simulink model "third"  (R2021b)
settings: Solver=VariableStepAuto  StartTime=0.0  StopTime=30.0  RelTol=1e-3
values from neighbouring files (symbols this model uses):
  Kd = 6    [analysis.m]    (also in params.m)
  KI = 6    [analysis.m]    (also in params.m)
  Km = 0.0642    [analysis.m]    (also in params.m)
  Kp = 0.6    [analysis.m]    (also in params.m)
  tau = 0.4    [analysis.m]    (also in params.m)
  wn = 3.8918    [analysis.m]    (also in params.m)
  zeta = 0.0044    [analysis.m]    (also in params.m = 0.0037)
settings Model: Creator=abomrar2  LastModifiedBy=abomrar2

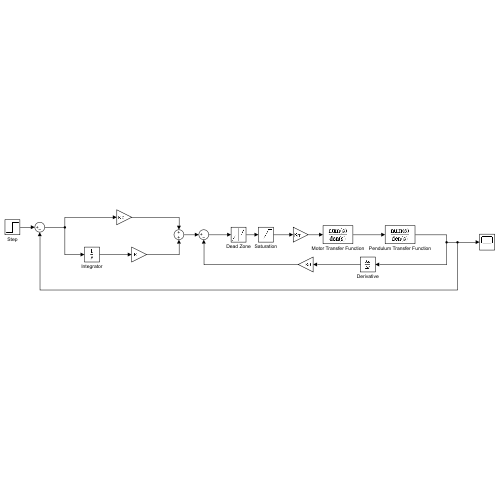
[thumbnail: Simulink's stored preview of the top-level diagram]
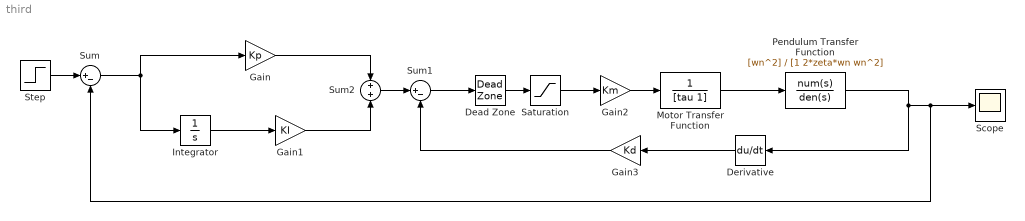
== system third ==
  Dead Zone : DeadZone  LowerValue=0  UpperValue=1.6534  SaturateOnIntegerOverflow=on
  Derivative : Derivative
  Gain : Gain  Gain=Kp
  Gain1 : Gain  Gain=KI
  Gain2 : Gain  Gain=Km
  Gain3 : Gain  Gain=Kd
  Integrator : Integrator
  Motor Transfer Function : TransferFcn  Denominator=[tau 1]
  Pendulum Transfer Function : TransferFcn  Numerator=[wn^2]  Denominator=[1 2*zeta*wn wn^2]
  Saturation : Saturate  UpperLimit=10  LowerLimit=-10
  Scope : Scope
  Step : Step  Time=0  After=0.5  SampleTime=0
  Sum : Sum  Inputs=|+-
  Sum1 : Sum  Inputs=|+-
  Sum2 : Sum  Inputs=+|+
  wires:
  Step/1 -> Sum/1
  Sum/1 -> Integrator/1, Gain/1
  Gain/1 -> Sum2/1
  Integrator/1 -> Gain1/1
  Gain1/1 -> Sum2/2
  Sum2/1 -> Sum1/1
  Sum1/1 -> Dead Zone/1
  Dead Zone/1 -> Saturation/1
  Saturation/1 -> Gain2/1
  Gain2/1 -> Motor Transfer Function/1
  Motor Transfer Function/1 -> Pendulum Transfer Function/1
  Pendulum Transfer Function/1 -> Derivative/1, Sum/2, Scope/1
  Derivative/1 -> Gain3/1
  Gain3/1 -> Sum1/2
